simulink model "Problem3"  (R2020b)
settings: Solver=VariableStepAuto  StartTime=0.0  StopTime=120  RelTol=1e-3
model workspace (MAT data in the model file):
  M = Simulink.Parameter
  M.Value = 1000
  M.DataType = 'auto'
  M.Dimensions = [1 1]
  Ts = Simulink.Parameter
  Ts.Value = 0.01
  Ts.DataType = 'auto'
  Ts.Dimensions = [1 1]
  b = Simulink.Parameter
  b.Value = 50
  b.DataType = 'auto'
  b.Dimensions = [1 1]
  kd = Simulink.Parameter
  kd.Value = 0
  kd.DataType = 'auto'
  kd.Dimensions = [1 1]
  ki = Simulink.Parameter
  ki.Value = 91.5
  ki.DataType = 'auto'
  ki.Dimensions = [1 1]
  kp = Simulink.Parameter
  kp.Value = 550
  kp.DataType = 'auto'
  kp.Dimensions = [1 1]
  u = Simulink.Parameter
  u.Value = 500
  u.DataType = 'auto'
  u.Dimensions = [1 1]
settings Model: Creator=HP  LastModifiedBy=HP

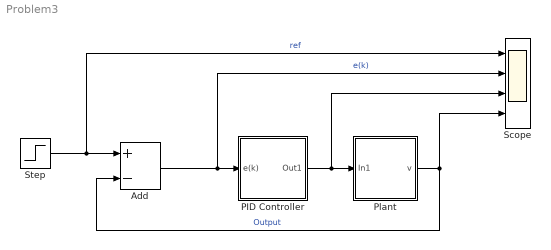
== system Problem3 ==
  Add : Sum  Inputs=+-
  PID Controller : Subsystem
  Plant : Subsystem
  Scope : Scope  NumInputPorts=4
  Step : Step  Time=0  After=u  SampleTime=0
  wires:
  Step/1 -> Scope/1, Add/1  "ref"
  Add/1 -> Scope/2, PID Controller/1(e(k))  "e(k)"
  PID Controller/1(Out1) -> Scope/3, Plant/1(In1)
  Plant/1(v) -> Scope/4, Add/2  "Output"

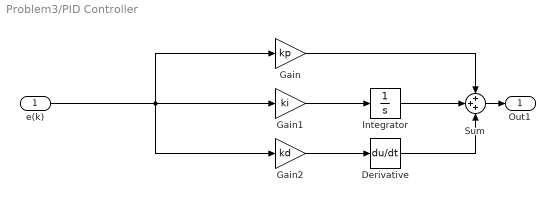
== system Problem3/PID Controller ==
  e(k) : Inport
  Derivative : Derivative
  Gain : Gain  Gain=kp
  Gain1 : Gain  Gain=ki
  Gain2 : Gain  Gain=kd
  Integrator : Integrator
  Sum : Sum  Inputs=+++
  Out1 : Outport
  wires:
  Gain/1 -> Sum/1
  Integrator/1 -> Sum/2
  Sum/1 -> Out1/1
  Gain2/1 -> Derivative/1
  e(k)/1 -> Gain/1, Gain2/1, Gain1/1
  Derivative/1 -> Sum/3
  Gain1/1 -> Integrator/1

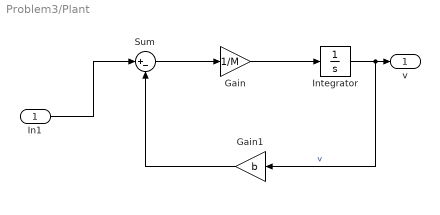
== system Problem3/Plant ==
  In1 : Inport
  Gain : Gain  Gain=1/M
  Gain1 : Gain  Gain=b
  Integrator : Integrator
  Sum : Sum  Inputs=|+-
  v : Outport
  wires:
  In1/1 -> Sum/1
  Sum/1 -> Gain/1
  Gain/1 -> Integrator/1
  Integrator/1 -> Gain1/1, v/1  "v"
  Gain1/1 -> Sum/2
